simulink library "threeTetherGroundStation_cl"  (R2018b)
settings: Solver=VariableStepAuto  StartTime=0.0  StopTime=10.0  RelTol=1e-3
libraries: vrlib x6, simulink x1, eulAng2RotMat_ul x1, massSpringDamper_ul x1
settings Model: Creator=M.Cobb  LastModifiedBy=M.Cobb

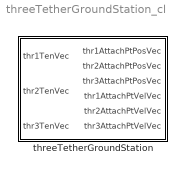
== system threeTetherGroundStation_cl ==
  threeTetherGroundStation : Subsystem  mask{fixed=0, J=0, b=0, thr1AttachPt=[0 1 0], thr2AttachPt=[1 0 0], thr3AttachPt=[0 -1 0], initAngPos=0, initAngVel=0}
      mask prompts: fixed "Free Spin Enable (==0 -> No Rotation, ~=0 -> Free Spinning)"; J "Rotational Inertia"; b "Damping coefficient"; thr1AttachPt "Tether 1"; thr2AttachPt "Tether 2"; thr3AttachPt "Tether 3"; initAngPos "Initial angle"; initAngVel "Inital angular velocity"
      mask DialogControl Container5 Prompt: Physical Parameters
      mask DialogControl Container3 Prompt: Tether attachment position vectors: platform frame
      mask DialogControl Container4 Prompt: Initial conditions

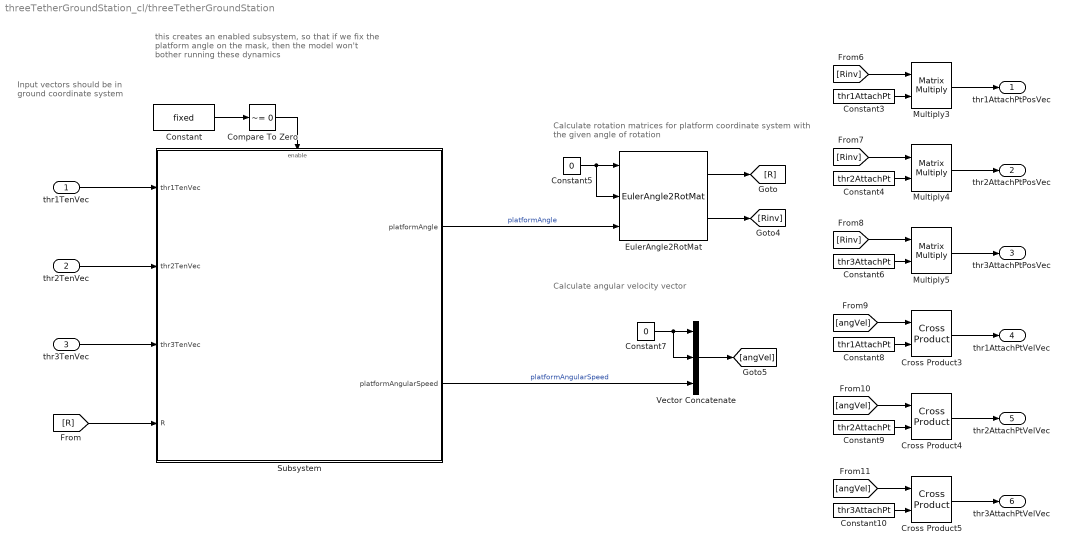
== system threeTetherGroundStation_cl/threeTetherGroundStation ==
  note: Calculate angular velocity vector
  note: Calculate rotation matrices for platform coordinate
      | system with the given angle of rotation
  note: Input vectors should be in
      | ground coordinate system
  note: this creates an enabled subsystem, so that if we fix
      | the platform angle on the mask,
      | then the model won't bother running these dynamics
  thr1TenVec : Inport
  thr2TenVec : Inport  Port=2
  thr3TenVec : Inport  Port=3
  Compare To Zero : simulink/Logic and Bit Operations/Compare To Zero  relop=~=  OutDataTypeStr=boolean
  Constant : Constant  Value=fixed
  Constant10 : Constant  Value=thr3AttachPt
  Constant3 : Constant  Value=thr1AttachPt
  Constant4 : Constant  Value=thr2AttachPt
  Constant5 : Constant  Value=0
  Constant6 : Constant  Value=thr3AttachPt
  Constant7 : Constant  Value=0
  Constant8 : Constant  Value=thr1AttachPt
  Constant9 : Constant  Value=thr2AttachPt
  Cross Product3 : vrlib/Utilities/Cross Product
      settings: SourceProductBaseCode=VR
  Cross Product4 : vrlib/Utilities/Cross Product
      settings: SourceProductBaseCode=VR
  Cross Product5 : vrlib/Utilities/Cross Product
      settings: SourceProductBaseCode=VR
  EulerAngle2RotMat : eulAng2RotMat_ul/EulerAngle2RotMat  SystemSampleTime=-1
  Multiply3 : Product  Multiplication=Matrix(*)
  Multiply4 : Product  Multiplication=Matrix(*)
  Multiply5 : Product  Multiplication=Matrix(*)
  Subsystem : Subsystem
      settings: MinAlgLoopOccurrences=on
  Vector Concatenate : Concatenate  NumInputs=3
  thr1AttachPtPosVec : Outport
  thr2AttachPtPosVec : Outport  Port=2
  thr3AttachPtPosVec : Outport  Port=3
  thr1AttachPtVelVec : Outport  Port=4
  thr2AttachPtVelVec : Outport  Port=5
  thr3AttachPtVelVec : Outport  Port=6
  wires:
  Constant5/1 -> EulerAngle2RotMat/2, EulerAngle2RotMat/1
  EulerAngle2RotMat/1 -> [R]
  EulerAngle2RotMat/2 -> [Rinv]
  [Rinv] -> Multiply3/1
  Constant3/1 -> Multiply3/2
  Multiply3/1 -> thr1AttachPtPosVec/1
  [Rinv] -> Multiply4/1
  [Rinv] -> Multiply5/1
  Multiply4/1 -> thr2AttachPtPosVec/1
  Multiply5/1 -> thr3AttachPtPosVec/1
  Constant4/1 -> Multiply4/2
  Constant6/1 -> Multiply5/2
  Constant7/1 -> Vector Concatenate/1, Vector Concatenate/2
  Vector Concatenate/1 -> [angVel]
  [angVel] -> Cross Product3/1
  Constant8/1 -> Cross Product3/2
  [angVel] -> Cross Product4/1
  [angVel] -> Cross Product5/1
  Constant9/1 -> Cross Product4/2
  Constant10/1 -> Cross Product5/2
  Cross Product3/1 -> thr1AttachPtVelVec/1
  Cross Product4/1 -> thr2AttachPtVelVec/1
  Cross Product5/1 -> thr3AttachPtVelVec/1
  thr1TenVec/1 -> Subsystem/1(thr1TenVec)
  thr2TenVec/1 -> Subsystem/2(thr2TenVec)
  thr3TenVec/1 -> Subsystem/3(thr3TenVec)
  Subsystem/1(platformAngle) -> EulerAngle2RotMat/3  "platformAngle"
  Subsystem/2(platformAngularSpeed) -> Vector Concatenate/3  "platformAngularSpeed"
  Constant/1 -> Compare To Zero/1
  Compare To Zero/1 -> Subsystem/Enable
  [R] -> Subsystem/4(R)

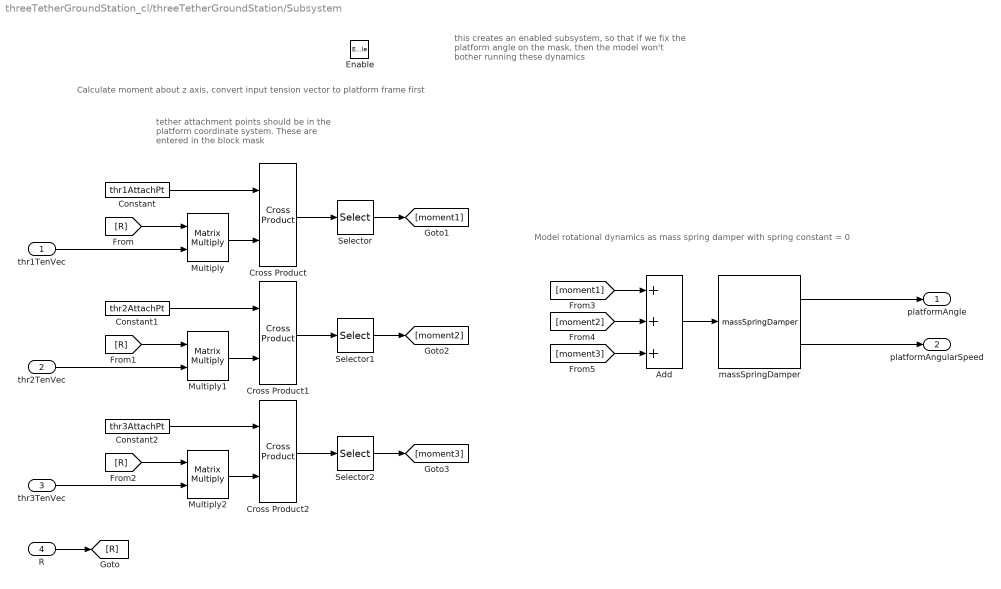
== system threeTetherGroundStation_cl/threeTetherGroundStation/Subsystem ==
  note: this creates an enabled subsystem, so that if we fix
      | the platform angle on the mask,
      | then the model won't bother running these dynamics
  note: Model rotational dynamics as mass spring damper with
      | spring constant = 0
  note: Calculate moment about z axis, convert input tension vector to platform frame first
  note: tether attachment points should be in
      | the platform coordinate system.  These
      | are entered in the block mask
  thr1TenVec : Inport
  thr2TenVec : Inport  Port=2
  thr3TenVec : Inport  Port=3
  R : Inport  Port=4
  Enable : EnablePort
  Add : Sum  Inputs=+++
  Constant : Constant  Value=thr1AttachPt
  Constant1 : Constant  Value=thr2AttachPt
  Constant2 : Constant  Value=thr3AttachPt
  Cross Product : vrlib/Utilities/Cross Product
      settings: SourceProductBaseCode=VR
  Cross Product1 : vrlib/Utilities/Cross Product
      settings: SourceProductBaseCode=VR
  Cross Product2 : vrlib/Utilities/Cross Product
      settings: SourceProductBaseCode=VR
  Multiply : Product  Multiplication=Matrix(*)
  Multiply1 : Product  Multiplication=Matrix(*)
  Multiply2 : Product  Multiplication=Matrix(*)
  Selector : Selector  InputPortWidth=3  IndexOptions=Index vector (dialog)  Indices=3  OutputSizes=1
  Selector1 : Selector  InputPortWidth=3  IndexOptions=Index vector (dialog)  Indices=3  OutputSizes=1
  Selector2 : Selector  InputPortWidth=3  IndexOptions=Index vector (dialog)  Indices=3  OutputSizes=1
  massSpringDamper : massSpringDamper_ul/massSpringDamper  m=J  b=b  k=0  x0=initAngPos  xDot0=initAngVel
  platformAngle : Outport  InitialOutput=initAngPos
  platformAngularSpeed : Outport  Port=2  InitialOutput=0
  wires:
  Selector1/1 -> [moment2]
  Constant/1 -> Cross Product/1
  [R] -> Multiply2/1
  [R] -> Multiply1/1
  [moment1] -> Add/1
  [R] -> Multiply/1
  [moment3] -> Add/3
  Cross Product2/1 -> Selector2/1
  Cross Product/1 -> Selector/1
  Constant2/1 -> Cross Product2/1
  Cross Product1/1 -> Selector1/1
  Constant1/1 -> Cross Product1/1
  Add/1 -> massSpringDamper/1
  Multiply/1 -> Cross Product/2
  Multiply1/1 -> Cross Product1/2
  Multiply2/1 -> Cross Product2/2
  Selector/1 -> [moment1]
  [moment2] -> Add/2
  Selector2/1 -> [moment3]
  massSpringDamper/1 -> platformAngle/1
  massSpringDamper/2 -> platformAngularSpeed/1
  thr3TenVec/1 -> Multiply2/2
  thr2TenVec/1 -> Multiply1/2
  thr1TenVec/1 -> Multiply/2
  R/1 -> [R]
